simulink model "Low_Shelf_2"  (R2024b)
settings: Solver=VariableStepAuto  StartTime=0.0  StopTime=10.0  RelTol=1e-3
settings Model: Creator=woutlyen  LastModifiedBy=woutlyen

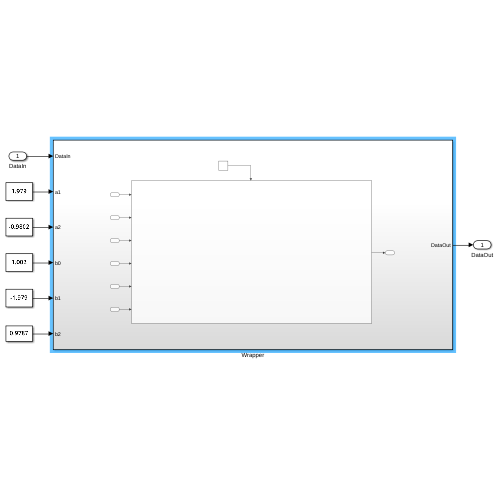
[thumbnail: Simulink's stored preview of the top-level diagram]
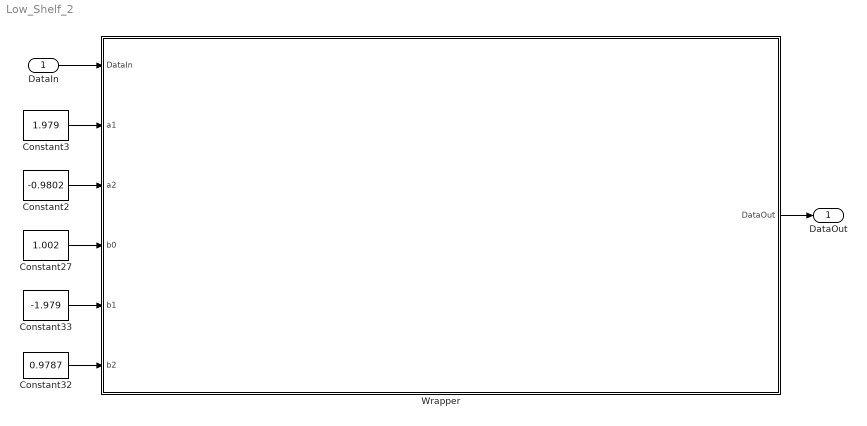
== system Low_Shelf_2 ==
  DataIn : Inport  OutDataTypeStr=fixdt(1,24,23)
  Constant2 : Constant  Value=-0.9802  OutDataTypeStr=fixdt(1,27,23)
  Constant27 : Constant  Value=1.002  OutDataTypeStr=fixdt(1,27,23)
  Constant3 : Constant  Value=1.979  OutDataTypeStr=fixdt(1,27,23)
  Constant32 : Constant  Value=0.9787  OutDataTypeStr=fixdt(1,27,23)
  Constant33 : Constant  Value=-1.979  OutDataTypeStr=fixdt(1,27,23)
  Wrapper : Subsystem
  DataOut : Outport
  wires:
  Wrapper/1(DataOut) -> DataOut/1
  Constant32/1 -> Wrapper/6(b2)
  Constant33/1 -> Wrapper/5(b1)
  Constant3/1 -> Wrapper/2(a1)
  Constant2/1 -> Wrapper/3(a2)
  Constant27/1 -> Wrapper/4(b0)
  DataIn/1 -> Wrapper/1(DataIn)

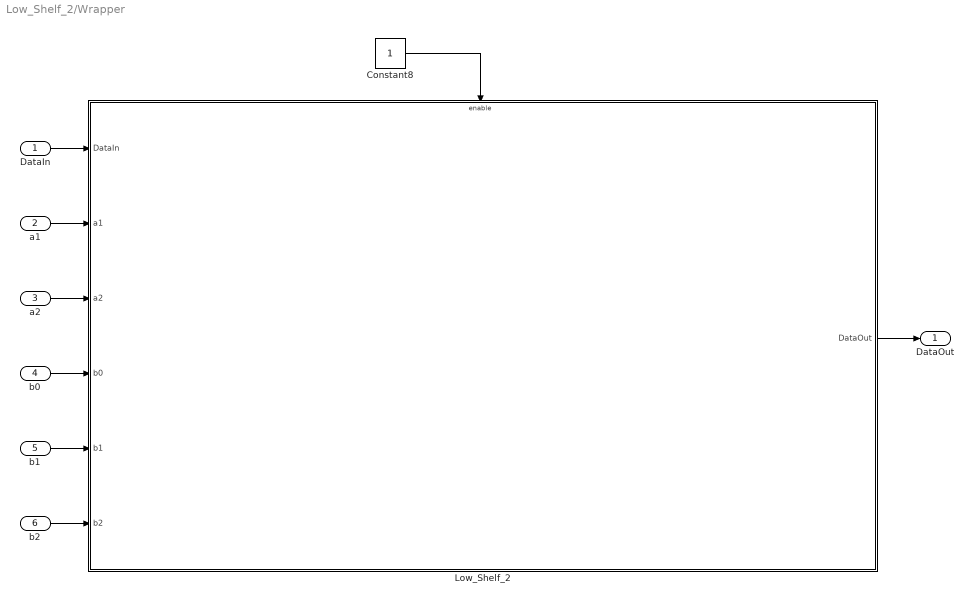
== system Low_Shelf_2/Wrapper ==
  DataIn : Inport
  a1 : Inport  Port=2
  a2 : Inport  Port=3
  b0 : Inport  Port=4
  b1 : Inport  Port=5
  b2 : Inport  Port=6
  Constant8 : Constant  OutDataTypeStr=boolean
  Low_Shelf_2 : Subsystem
  DataOut : Outport
  wires:
  b2/1 -> Low_Shelf_2/6(b2)
  a1/1 -> Low_Shelf_2/2(a1)
  b0/1 -> Low_Shelf_2/4(b0)
  Low_Shelf_2/1(DataOut) -> DataOut/1
  DataIn/1 -> Low_Shelf_2/1(DataIn)
  a2/1 -> Low_Shelf_2/3(a2)
  Constant8/1 -> Low_Shelf_2/Enable
  b1/1 -> Low_Shelf_2/5(b1)

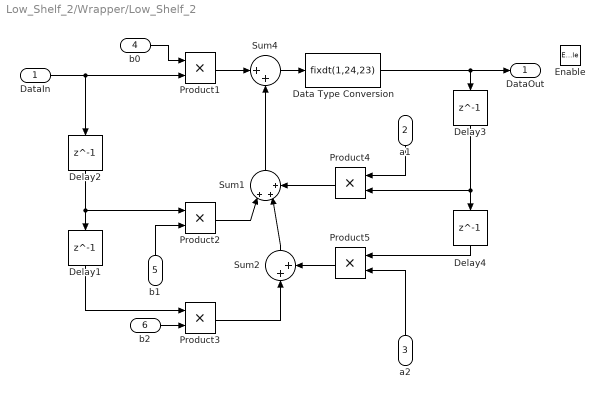
== system Low_Shelf_2/Wrapper/Low_Shelf_2 ==
  DataIn : Inport
  a1 : Inport  Port=2
  a2 : Inport  Port=3
  b0 : Inport  Port=4
  b1 : Inport  Port=5
  b2 : Inport  Port=6
  Enable : EnablePort
  Data Type Conversion : DataTypeConversion  OutDataTypeStr=fixdt(1,24,23)  SaturateOnIntegerOverflow=off  RndMeth=Floor
  Delay{1..4} (4 alike) : Delay  DelayLength=1  InitialCondition=0
  Product{1..5} (5 alike) : Product  OutDataTypeStr=fixdt(1,27,23)
  Sum1 : Sum  Inputs=|+++
  Sum2 : Sum  Inputs=|++
  Sum4 : Sum  Inputs=|++
  DataOut : Outport  VectorParamsAs1DForOutWhenUnconnected=off
  wires:
  Sum2/1 -> Sum1/2
  Delay4/1 -> Product5/1
  a2/1 -> Product5/2
  b2/1 -> Product3/2
  Delay2/1 -> Product2/1, Delay1/1
  Delay1/1 -> Product3/1
  a1/1 -> Product4/1
  Sum1/1 -> Sum4/2
  b0/1 -> Product1/1
  Product3/1 -> Sum2/1
  Product4/1 -> Sum1/3
  Delay3/1 -> Product4/2, Delay4/1
  b1/1 -> Product2/2
  Sum4/1 -> Data Type Conversion/1
  Product2/1 -> Sum1/1
  Product1/1 -> Sum4/1
  DataIn/1 -> Product1/2, Delay2/1
  Product5/1 -> Sum2/2
  Data Type Conversion/1 -> DataOut/1, Delay3/1
